simulink model "lab5"  (R2019a)
settings: Solver=VariableStepAuto  StartTime=0.0  StopTime=10.0  RelTol=1e-3
settings Model: Creator=sumli  LastModifiedBy=sumli

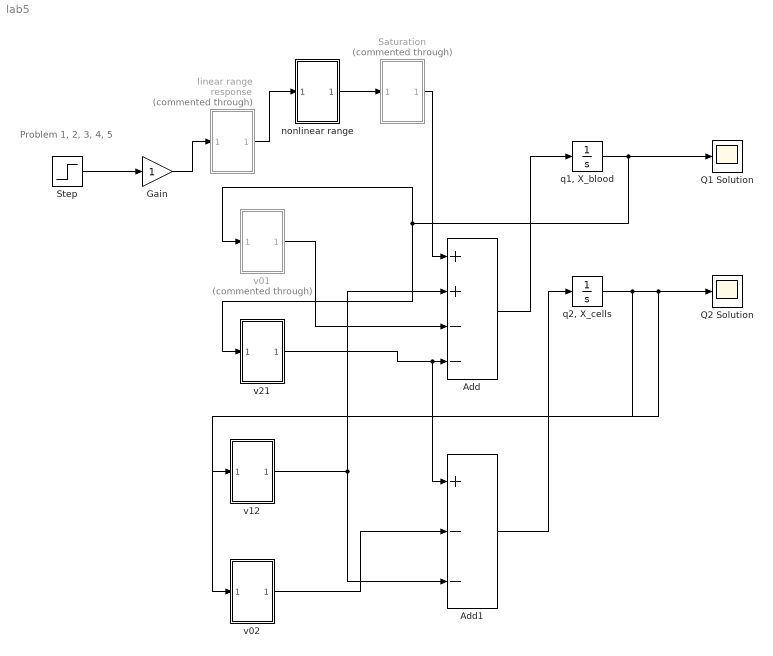
== system lab5 ==
  note: Problem 1, 2, 3, 4, 5
  Add : Sum  Inputs=++--
  Add1 : Sum  Inputs=+--
  Gain : Gain
  Q1 Solution : Scope
  Q2 Solution : Scope
  Saturation : Subsystem  Commented=through
  Step : Step  Time=10  Before=1  SampleTime=10
  linear range response : Subsystem  Commented=through
  nonlinear range : Subsystem
  "q1, X_blood" : Integrator
  "q2, X_cells" : Integrator
  v01 : Subsystem  Commented=through
  v02 : Subsystem
  v12 : Subsystem
  v21 : Subsystem
  wires:
  "q1, X_blood"/1 -> v21/1(In1), v01/1(In1), Q1 Solution/1
  "q2, X_cells"/1 -> v12/1(In1), Q2 Solution/1, v02/1(In1)
  Add/1 -> "q1, X_blood"/1
  Add1/1 -> "q2, X_cells"/1
  v12/1(Out1) -> Add1/3, Add/2
  v01/1(Out1) -> Add/3
  v21/1(Out1) -> Add1/1, Add/4
  v02/1(Out1) -> Add1/2
  Step/1 -> Gain/1
  Gain/1 -> linear range response/1(In1)
  linear range response/1(Out1) -> nonlinear range/1(In1)
  nonlinear range/1(Out1) -> Saturation/1(In1)
  Saturation/1(Out1) -> Add/1

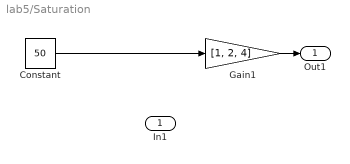
== system lab5/Saturation ==
  In1 : Inport
  Constant : Constant  Value=50
  Gain1 : Gain  Gain=[1, 2, 4]
  Out1 : Outport
  wires:
  Gain1/1 -> Out1/1
  Constant/1 -> Gain1/1

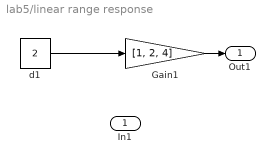
== system lab5/linear range response ==
  In1 : Inport
  Gain1 : Gain  Gain=[1, 2, 4]
  d1 : Constant  Value=2
  Out1 : Outport
  wires:
  Gain1/1 -> Out1/1
  d1/1 -> Gain1/1

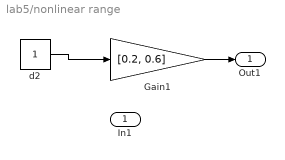
== system lab5/nonlinear range ==
  In1 : Inport
  Gain1 : Gain  Gain=[0.2, 0.6]
  d2 : Constant
  Out1 : Outport
  wires:
  Gain1/1 -> Out1/1
  d2/1 -> Gain1/1

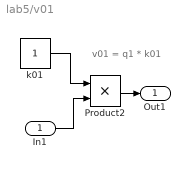
== system lab5/v01 ==
  note: v01 = q1 * k01
  In1 : Inport
  Product2 : Product
  k01 : Constant
  Out1 : Outport
  wires:
  In1/1 -> Product2/2
  Product2/1 -> Out1/1
  k01/1 -> Product2/1

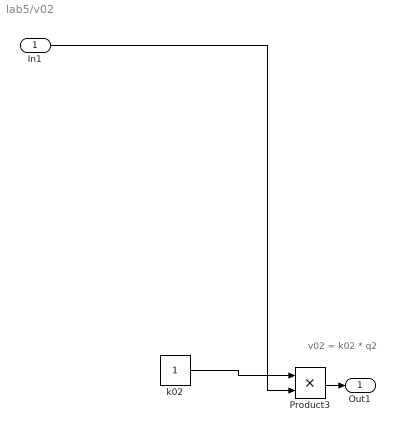
== system lab5/v02 ==
  note: v02 = k02 * q2
  In1 : Inport
  Product3 : Product
  k02 : Constant
  Out1 : Outport
  wires:
  Product3/1 -> Out1/1
  In1/1 -> Product3/2
  k02/1 -> Product3/1

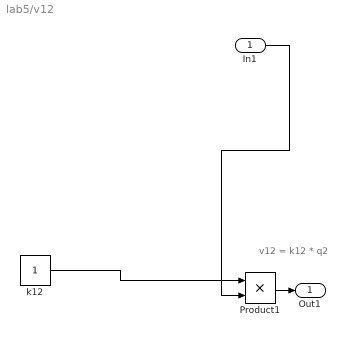
== system lab5/v12 ==
  note: v12 = k12 * q2
  In1 : Inport
  Product1 : Product
  k12 : Constant
  Out1 : Outport
  wires:
  In1/1 -> Product1/2
  Product1/1 -> Out1/1
  k12/1 -> Product1/1

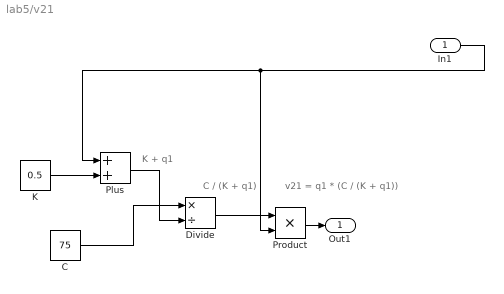
== system lab5/v21 ==
  note: C / (K + q1)
  note: K + q1
  note: v21 = q1 * (C / (K + q1))
  In1 : Inport
  C : Constant  Value=75
  Divide : Product  Inputs=*/
  K : Constant  Value=0.5
  Plus : Sum
  Product : Product
  Out1 : Outport
  wires:
  Divide/1 -> Product/1
  Plus/1 -> Divide/2
  C/1 -> Divide/1
  K/1 -> Plus/2
  Product/1 -> Out1/1
  In1/1 -> Product/2, Plus/1
